simulink model "xc8gyz2"  (R2022a)
settings: Solver=VariableStepAuto  StartTime=0.0  StopTime=80  RelTol=1e-3
settings Model: Creator=dell  LastModifiedBy=dell

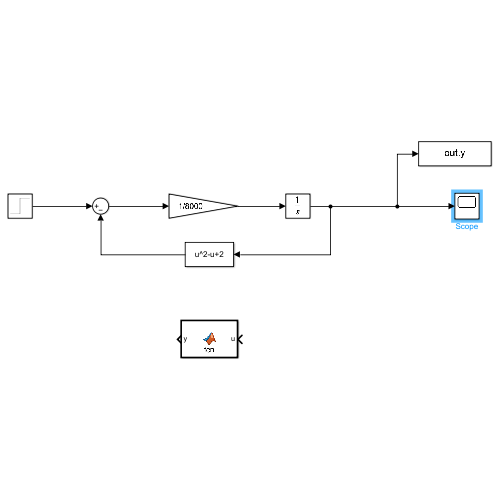
[thumbnail: Simulink's stored preview of the top-level diagram]
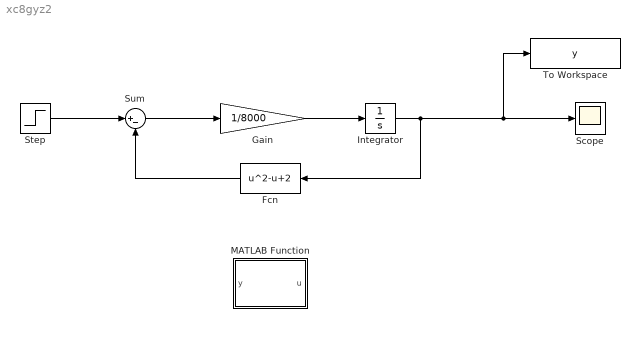
== system xc8gyz2 ==
  Fcn : Fcn  Expr=u^2-u+2
  Gain : Gain  Gain=1/8000
  Integrator : Integrator
  MATLAB Function : MATLAB Function  TreatAsAtomicUnit=on
  Scope : Scope
  Step : Step  After=150000  SampleTime=0
  Sum : Sum  Inputs=|+-
  To Workspace : ToWorkspace  VariableName=y  SaveFormat=Timeseries  SampleTime=-1
  wires:
  Step/1 -> Sum/1
  Sum/1 -> Gain/1
  Gain/1 -> Integrator/1
  Integrator/1 -> Fcn/1, To Workspace/1, Scope/1
  Fcn/1 -> Sum/2

== matlab function xc8gyz2/MATLAB Function ==
  data: u input; y output
function y = fcn(u)
y = u^2-u+2;
